simulink model "dc_motor"  (R2014a)
settings: Solver=ode45  StartTime=0.0  StopTime=10.0  RelTol=1e-3
values from neighbouring files (symbols this model uses):
  b = output_rules(output_tags(4))    [fuzzy_inference.m]
undefined symbols (not defined in the file or in its folder): J, K, L, R
libraries: simulink x1, simulink_extras x1
settings Model: Creator=krish  LastModifiedBy=krish

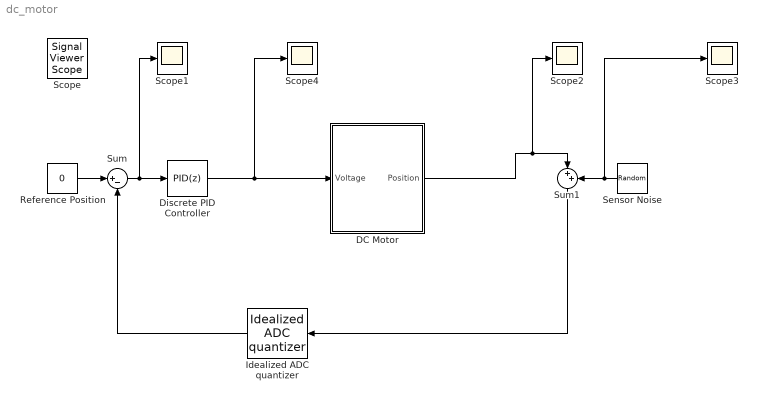
== system dc_motor ==
  DC Motor : Subsystem
  Discrete PID Controller : simulink/Continuous/PID Controller  Controller=PID  TimeDomain=Discrete-time  SampleTime=1  IntegratorMethod=Forward Euler  FilterMethod=Forward Euler  Form=Parallel  P=1  I=1  D=0  N=100  InitialConditionSource=internal  InitialConditionForIntegrator=0  InitialConditionForFilter=0  ExternalReset=none  LimitOutput=off  UpperSaturationLimit=inf  LowerSaturationLimit=-inf  LinearizeAsGain=off  AntiWindupMode=none  Kb=1  TrackingMode=off  Kt=1  PParamMin=[]  PParamMax=[]  IParamMin=[]  IParamMax=[]  DParamMin=[]  DParamMax=[]  NParamMin=[]  NParamMax=[]  KbParamMin=[]  KbParamMax=[]  KtParamMin=[]  KtParamMax=[]  POutMin=[]  POutMax=[]  IOutMin=[]  IOutMax=[]  DOutMin=[]  DOutMax=[]  NOutMin=[]  NOutMax=[]  KbOutMin=[]  KbOutMax=[]  KtOutMin=[]  KtOutMax=[]  IntegratorOutMin=[]  IntegratorOutMax=[]  FilterOutMin=[]  FilterOutMax=[]  SumOutMin=[]  SumOutMax=[]  SumI1OutMin=[]  SumI1OutMax=[]  SumI2OutMin=[]  SumI2OutMax=[]  SumI3OutMin=[]  SumI3OutMax=[]  SumDOutMin=[]  SumDOutMax=[]  SaturationOutMin=[]  SaturationOutMax=[]  IntegratorContinuousStateAttributes=''  IntegratorStateMustResolveToSignalObject=off  IntegratorRTWStateStorageClass=Auto  FilterContinuousStateAttributes=''  FilterStateMustResolveToSignalObject=off  FilterRTWStateStorageClass=Auto
  Idealized ADC quantizer : simulink_extras/Additional Discrete/Idealized ADC quantizer  NumberOfConverterBits=12  Vmin=0  Vmax=5  OutputDataType=int16  OutputNegativeValues=off
  Reference Position : Constant  Value=0
  Scope{1..4} (4 alike) : Scope
      Scope2 settings: TimeRange=10
      Scope3 settings: SaveName=ScopeData2
      Scope4 settings: SaveName=ScopeData3
  Sensor Noise : RandomNumber  SampleTime=0.1
  Sum : Sum  Inputs=|+-
  Sum1 : Sum  Inputs=|++
  Scope : SignalViewerScope  IOType=viewer  RefreshTime=0.035000
  wires:
  DC Motor/1(Position) -> Scope2/1, Sum1/1
  Idealized ADC quantizer/1 -> Sum/2
  Reference Position/1 -> Sum/1
  Sum/1 -> Scope1/1, Discrete PID Controller/1
  Discrete PID Controller/1 -> Scope4/1, DC Motor/1(Voltage)
  Sum1/1 -> Idealized ADC quantizer/1
  Sensor Noise/1 -> Scope3/1, Sum1/2

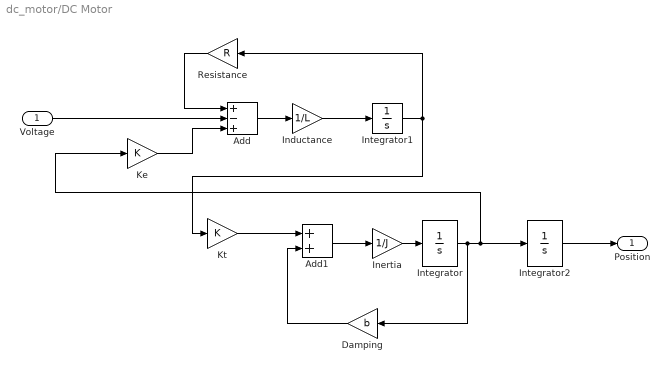
== system dc_motor/DC Motor ==
  Voltage : Inport
  " Inductance" : Gain  Gain=1/L
  Add : Sum  Inputs=+-+
  Add1 : Sum
  Damping : Gain  Gain=b
  Inertia : Gain  Gain=1/J
  Integrator : Integrator
  Integrator1 : Integrator
  Integrator2 : Integrator
  "Ke " : Gain  Gain=K
  "Kt " : Gain  Gain=K
  "Resistance " : Gain  Gain=R
  Position : Outport
  wires:
  "Resistance "/1 -> Add/1
  Add1/1 -> Inertia/1
  Voltage/1 -> Add/2
  "Ke "/1 -> Add/3
  Integrator/1 -> Integrator2/1, "Ke "/1, Damping/1
  Integrator2/1 -> Position/1
  Inertia/1 -> Integrator/1
  Damping/1 -> Add1/2
  "Kt "/1 -> Add1/1
  " Inductance"/1 -> Integrator1/1
  Add/1 -> " Inductance"/1
  Integrator1/1 -> "Kt "/1, "Resistance "/1
